simulink subsystem "Cycler"  (R2022a)
settings: Solver=VariableStepAuto  StartTime=0.0  StopTime=10.0  RelTol=1e-3
undefined symbols (not defined in the file): Neg, Pos
libraries: fl_lib x8, nesl_utility x8, ee_lib x2
settings Model: Creator=mmarq  LastModifiedBy=mmarq

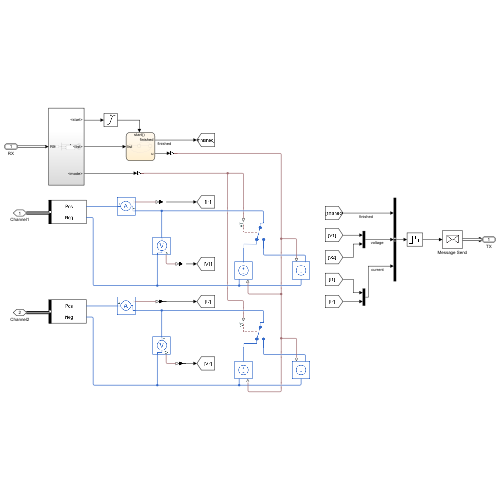
[thumbnail: Simulink's stored preview of the top-level diagram]
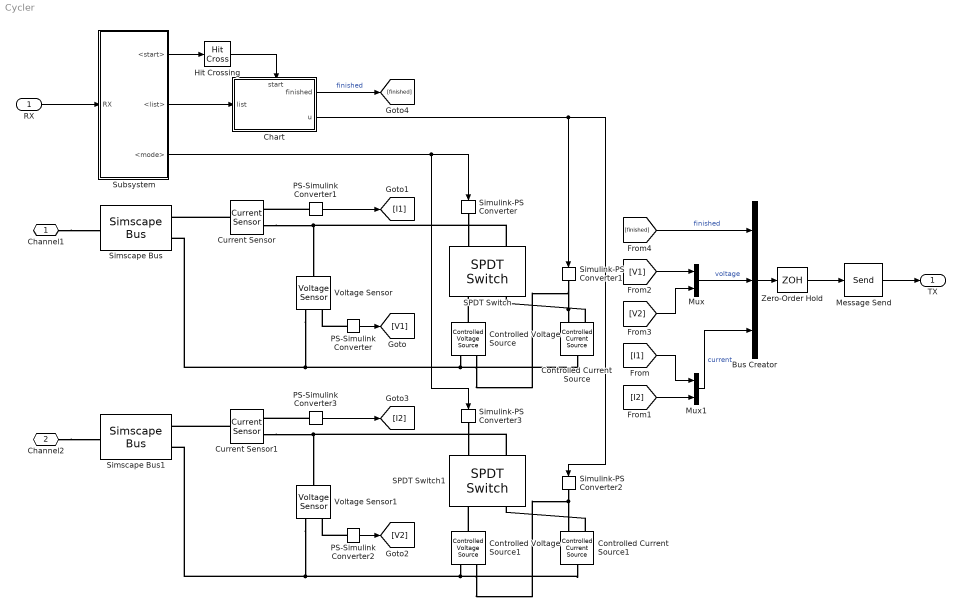
== system Cycler ==
  RX : Inport  OutputPortMessageModes=m  OutDataTypeStr=Bus: CyclerCmd
  Bus Creator : BusCreator  Inputs=3  OutDataTypeStr=Bus: CyclerData  NonVirtualBus=on
  Chart : Stateflow chart  TreatAsAtomicUnit=on
      settings: PortSchema="{\"entries\":[{\"content\":{\"sides\":[{\"content\":{\"connectorIds\":[\"In1\"]},\"type\":\"ConnectorPlacement.EquallySpacedRectSide\",\"uuid\":\"4ed828f0-1ac9-4dcc-9380-eef59d4566e8\"},{\"content\":{\"connectorIds\":[\"Out1\",\"Out2\"],\"side\":\"RIGHT\"},\"type\":\"ConnectorPlacement.EquallySpacedRectSide\",\"uuid\":\"89d19431-af69-4c25-9773-8ef87ef26c35\"},{\"content\":{\"connectorIds\":[\"In2\"],\"side\":\"TOP\"},\"type\":\"ConnectorPlacement.EquallySpacedRectSide\",\"uuid\":\"16b2249e-20d7-4791-ad8a-e9d093ae3788\"}]},\"type\":\"ConnectorPlacement.EquallySpacedConnector\",\"uuid\":\"4997d404-275d-4b55-9693-2b863566ce67\"}],\"packageUris\":[\"http://schema.mathworks.com/mf0/Connector/R2020b\"],\"version\":\"1.0\"}"
  Controlled Current Source : fl_lib/Electrical/Electrical Sources/Controlled Current Source
      settings: SourceProductBaseCode=PW,SS,VE
  Controlled Current Source1 : fl_lib/Electrical/Electrical Sources/Controlled Current Source
      settings: SourceProductBaseCode=PW,SS,VE
  Controlled Voltage Source : fl_lib/Electrical/Electrical Sources/Controlled Voltage Source
      settings: SourceProductBaseCode=PW,SS,VE
  Controlled Voltage Source1 : fl_lib/Electrical/Electrical Sources/Controlled Voltage Source
      settings: SourceProductBaseCode=PW,SS,VE
  Current Sensor : fl_lib/Electrical/Electrical Sensors/Current Sensor
      settings: SourceProductBaseCode=PW,SS,VE
  Current Sensor1 : fl_lib/Electrical/Electrical Sensors/Current Sensor
      settings: SourceProductBaseCode=PW,SS,VE
  Hit Crossing : HitCross  HitCrossingDirection=rising
  Message Send : Send  OutputPortMessageModes=m
  Mux : Mux  Inputs=2
  Mux1 : Mux  Inputs=2
  PS-Simulink Converter{,1..3} (4 alike) : nesl_utility/PS-Simulink Converter  PhysicalDomain=network_engine_domain  SubClassName=ps_output  LeftPortType=input  RightPortType=output  PseudoPeriodic=off  Frequencies=[]  VectorFormat=inherit  Unit=inherit  AffineConversion=off
      settings: SourceProductBaseCode=SS,PW,VE
  SPDT Switch : ee_lib/Switches & Breakers/SPDT Switch  R_closed=0.01 Ohm  G_open=1e-6 S  Threshold=0.5 V  Width=0 V  model_dynamics=0  t_on=1e-3 s  t_off=1e-3 s  initial_vT=0 V
      settings: SourceProductBaseCode=PS
  SPDT Switch1 : ee_lib/Switches & Breakers/SPDT Switch  R_closed=0.01 Ohm  G_open=1e-6 S  Threshold=0.5 V  Width=0 V  model_dynamics=0  t_on=1e-3 s  t_off=1e-3 s  initial_vT=0 V
      settings: SourceProductBaseCode=PS
  Simscape Bus : SimscapeBus  HierarchyStrings=Pos;Neg
  Simscape Bus1 : SimscapeBus  HierarchyStrings=Pos;Neg
  Simulink-PS Converter{,1..3} (4 alike) : nesl_utility/Simulink-PS Converter  PhysicalDomain=network_engine_domain  SubClassName=ps_input  LeftPortType=input  RightPortType=output  PseudoPeriodic=off  Frequencies=[]  NoiseDistribution=none  NoiseParameters=[]  Unit=1  AffineConversion=off  FilteringAndDerivatives=provide  SimscapeFilterOrder=1  InputFilterTimeConstant=0.001  UdotUserProvided=0
      settings: SourceProductBaseCode=SS,PW,VE
  Subsystem : Subsystem
  Voltage Sensor : fl_lib/Electrical/Electrical Sensors/Voltage Sensor
      settings: SourceProductBaseCode=PW,SS,VE
  Voltage Sensor1 : fl_lib/Electrical/Electrical Sensors/Voltage Sensor
      settings: SourceProductBaseCode=PW,SS,VE
  Zero-Order Hold : ZeroOrderHold  SampleTime=1e-3
  Channel1 : PMIOPort  Side=Left
  Channel2 : PMIOPort  Port=2  Side=Left
  TX : Outport  InputPortMessageModes=m  OutDataTypeStr=Bus: CyclerData
  wires:
  Mux/1 -> Bus Creator/2  "voltage"
  [V2] -> Mux/2
  Zero-Order Hold/1 -> Message Send/1
  [I2] -> Mux1/2
  [V1] -> Mux/1
  RX/1 -> Subsystem/1(RX)
  Chart/1(finished) -> [finished]  "finished"
  Bus Creator/1 -> Zero-Order Hold/1
  Mux1/1 -> Bus Creator/3  "current"
  [finished] -> Bus Creator/1  "finished"
  [I1] -> Mux1/1
  Subsystem/1(<start>) -> Hit Crossing/1
  Hit Crossing/1 -> Chart/2(start)
  Message Send/1 -> TX/1
  Subsystem/2(<list>) -> Chart/1(list)
  Subsystem/3(<mode>) -> Simulink-PS Converter/1, Simulink-PS Converter3/1
  Chart/2(u) -> Simulink-PS Converter1/1, Simulink-PS Converter2/1
  PS-Simulink Converter/1 -> [V1]
  PS-Simulink Converter1/1 -> [I1]
  PS-Simulink Converter3/1 -> [I2]
  PS-Simulink Converter2/1 -> [V2]
  connections:
  Controlled Current Source/LConn1 -- Simscape Bus/LConn2 -- Voltage Sensor/RConn2 -- Controlled Voltage Source/RConn2
  Current Sensor/RConn2 -- SPDT Switch/LConn2 -- Voltage Sensor/LConn1
  Controlled Current Source1/LConn1 -- Voltage Sensor1/RConn2 -- Simscape Bus1/LConn2 -- Controlled Voltage Source1/RConn2
  Current Sensor1/RConn2 -- SPDT Switch1/LConn2 -- Voltage Sensor1/LConn1
  Controlled Current Source/RConn1 -- Controlled Voltage Source/RConn1 -- Simulink-PS Converter1/RConn1
  Simulink-PS Converter2/RConn1 -- Controlled Voltage Source1/RConn1 -- Controlled Current Source1/RConn1
  Simulink-PS Converter/RConn1 -- SPDT Switch/LConn1
  Channel1/RConn1 -- Simscape Bus/RConn1
  PS-Simulink Converter1/LConn1 -- Current Sensor/RConn1
  Current Sensor/LConn1 -- Simscape Bus/LConn1
  PS-Simulink Converter/LConn1 -- Voltage Sensor/RConn1
  Controlled Voltage Source/LConn1 -- SPDT Switch/RConn1
  Controlled Current Source/RConn2 -- SPDT Switch/RConn2
  Controlled Current Source1/RConn2 -- SPDT Switch1/RConn2
  Current Sensor1/LConn1 -- Simscape Bus1/LConn1
  PS-Simulink Converter2/LConn1 -- Voltage Sensor1/RConn1
  PS-Simulink Converter3/LConn1 -- Current Sensor1/RConn1
  Channel2/RConn1 -- Simscape Bus1/RConn1
  Controlled Voltage Source1/LConn1 -- SPDT Switch1/RConn1
  Simulink-PS Converter3/RConn1 -- SPDT Switch1/LConn1

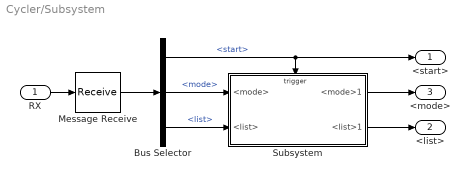
== system Cycler/Subsystem ==
  RX : Inport  OutDataTypeStr=Bus: CyclerCmd
  Bus Selector : BusSelector  OutputSignals=start,mode,list
  Message Receive : Receive  InputPortMessageModes=m  UseInternalQueue=off  QueueOverwriting=on  QueueLength=1  ValueSourceWhenQueueIsEmpty=Use initial value
  Subsystem : Subsystem
  <start> : Outport
  <list> : Outport  Port=2
  <mode> : Outport  Port=3
  wires:
  Message Receive/1 -> Bus Selector/1
  RX/1 -> Message Receive/1
  Bus Selector/1 -> <start>/1, Subsystem/Trigger  "<start>"
  Bus Selector/2 -> Subsystem/1(<mode>)  "<mode>"
  Bus Selector/3 -> Subsystem/2(<list>)  "<list>"
  Subsystem/1(<mode>1) -> <mode>/1
  Subsystem/2(<list>1) -> <list>/1

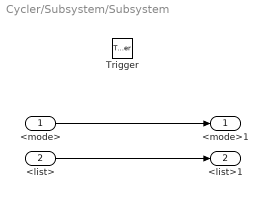
== system Cycler/Subsystem/Subsystem ==
  <mode> : Inport
  <list> : Inport  Port=2
  Trigger : TriggerPort  VariantControl=(inherit)  PortDimensions=1
  <mode>1 : Outport
  <list>1 : Outport  Port=2
  wires:
  <list>/1 -> <list>1/1
  <mode>/1 -> <mode>1/1

== stateflow chart Cycler/Chart ==
  settings: sampleTime=0.001  executeAtInitialization=1
  state Idle
    idx = 1;
    u = 0;
  state setOutput
    u=values(idx,1);
  state Next
  Next -> setOutput [order 1] : [idx<100]{idx=idx+1;}
  (default) -> Idle
  Idle -> setOutput : [start==1]{values=list;}
  setOutput -> Next : [after(values(idx,2),sec)]
  Next -> Idle [order 2] : {finished=1;}
  data: finished output; list input; u output; idx local; values local; start input
